simulink model "consigna_5_2"  (R2024b)
settings: Solver=ode45  StartTime=0.0  StopTime=600  FixedStep=1/39789  MaxStep=1e-1  RelTol=1e-5
InitFcn:
  | parametros
values from neighbouring files (symbols this model uses):
  A_corrientes = [0 1; -omega_n_corrientes^2 -2*omega_n_corrientes]    [parametros.m]
  A_inversor = [0 1; -omega_n_inversor^2 -2*omega_n_inversor]    [parametros.m]
  A_posicion = [0 1; -omega_n_posicion^2 -2*omega_n_posicion]    [parametros.m]
  A_temp = -1/20    (= -0.05)    [parametros.m]
  alpha_cu = 3.9 *10^-3    (= 0.0039)    [parametros.m]
  B_corrientes = [0; omega_n_corrientes^2]    [parametros.m]
  B_inversor = [0; omega_n_inversor^2]    [parametros.m]
  b_l = 0.1    [parametros.m]
  b_m = 1.5 * 10^-5    (= 1.5e-05)    [parametros.m]
  B_posicion = [0; omega_n_posicion^2]    [parametros.m]
  B_temp = 1/20    (= 0.05)    [parametros.m]
  ba = J_eq*n*omega_pos    (= 0.0395694444444)    [parametros.m]
  C_corrientes = [1 0]    [parametros.m]
  C_inversor = [1 0]    [parametros.m]
  C_posicion = [1 0]    [parametros.m]
  C_temp = 1    [parametros.m]
  C_ts = 0.818    [parametros.m]
  J_l = (m*l_cm^2 + J_cm) + (m_l * l_l^2)    (= 0.0833)    [parametros.m]
  J_m = 1.4 * 10^-5    (= 1.4e-05)    [parametros.m]
  K_e_int = 3200 ^3    (= 32768000000)    [parametros.m]
  K_e_omega = 3*3200^2    (= 30720000)    [parametros.m]
  K_e_theta = 9600    [parametros.m]
  k_l = m * g * l_cm + m_l * g * l_l    (= 2.4516625)    [parametros.m]
  Ksa = J_eq*n*(omega_pos^2)    (= 31.6555555556)    [parametros.m]
  Ksia = J_eq*(omega_pos^3)    (= 10129.7777778)    [parametros.m]
  L_d = 6.6 * 10^-3    (= 0.0066)    [parametros.m]
  L_ls = 0.8 * 10^-3    (= 0.0008)    [parametros.m]
  L_q = 5.8 * 10^-3    (= 0.0058)    [parametros.m]
  lambda_m = 0.016    [parametros.m]
  P_p = 3    [parametros.m]
  r = 120    [parametros.m]
  R_s_40 = 1.02    [parametros.m]
  R_ts_amb = 146.7    [parametros.m]
  T_sample = 1/f_sample    (= 4.53514739229e-05)    [parametros.m]
  Temp_s_ref = 20    [parametros.m]
  tm = X(1)    [parametros.m]
  tr = X(2)    [parametros.m]
  w1 = 2*pi*r/5    (= 150.796447372)    [parametros.m]
  x0_corrientes = [0;0]    [parametros.m]
  x0_inversor = [0;0]    [parametros.m]
  x0_posicion = [0; 0]    [parametros.m]
  x0_temp = 25    [parametros.m]
libraries: simulink x23, dspsigops x6
(part 5 of 5)

== system consigna_5_2/Subsystem/5.2.6/Subsistema físico no lineal ==
  note: Retroalimentación natural del torque gravitacional
  T_per : Inport
  v_as : Inport  Port=2
  v_bs : Inport  Port=3
  v_cs : Inport  Port=4
  Tº_amb : Inport  Port=5
  Gain : Gain  Gain=P_p
  Gain1 : Gain  Gain=1/r
  Gain2 : Gain  Gain=k_l
  Mux : Mux  Inputs=3
  Scope : Scope
  Sin : Trigonometry
  Subsistema electromagnético : Subsystem
      settings: PortSchema="{\"entries\":[{\"content\":{\"sides\":[{\"content\":{\"connectorIds\":[\"In1\",\"In2\",\"In3\",\"In4\"]},\"type\":\"ConnectorPlacement.EquallySpacedRectSide\",\"uuid\":\"c9fae60f-a644-4c7d-9a50-e330e891aba8\"},{\"content\":{\"connectorIds\":[\"Out1\",\"Out2\",\"Out3\",\"Out4\"],\"side\":\"RIGHT\"},\"type\":\"ConnectorPlacement.EquallySpacedRectSide\",\"uuid\":\"1bd25713-f5e9-4106-83eb-fb9f8a30d88e\"},{\"content\":{\"connectorIds\":[\"In5\"],\"side\":\"TOP\"},\"type\":\"ConnectorPlacement.EquallySpacedRectSide\",\"uuid\":\"c2f005dd-e04f-426d-b804-ce475aa5422d\"}]},\"type\":\"ConnectorPlacement.EquallySpacedConnector\",\"uuid\":\"9bdc4406-fcef-47cb-a5c0-d4f33f547a91\"}],\"packageUris\":[\"http://schema.mathworks.com/mf0/Connector/R2020b\"],\"version\":\"1.0\"}"
  Subsistema mecánico completo : Subsystem
  Subsistema térmico : Subsystem
  Sum : Sum  Inputs=++|
  TD_PARK : MATLAB Function  TreatAsAtomicUnit=on
  TI_PARK : MATLAB Function  TreatAsAtomicUnit=on
  theta_m : Outport
  T_s : Outport  Port=2
  i_abcs : Outport  Port=3
  omega_m : Outport  Port=4
  T_m : Outport  Port=5
  T_l : Outport  Port=6
  wires:
  Subsistema electromagnético/4(T_m) -> T_m/1, Subsistema mecánico completo/1(T_m)
  Subsistema electromagnético/3(i_0s) -> Subsistema térmico/3(i_0s^r), TI_PARK/3(f0s)
  Subsistema mecánico completo/2(omega_m(t)) -> Subsistema electromagnético/5(omega_m), Scope/1, omega_m/1
  Subsistema electromagnético/1(i_qs^r) -> Subsistema térmico/1(i_qs^r), TI_PARK/1(fqs)
  Subsistema electromagnético/2(i_ds^r) -> Subsistema térmico/2(i_ds^r), TI_PARK/2(fds)
  Sum/1 -> T_l/1, Subsistema mecánico completo/2(T_l)  "T_l"
  TD_PARK/1(fqs) -> Subsistema electromagnético/1(v_qs^r)
  Tº_amb/1 -> Subsistema térmico/4(Tº_amb)
  Mux/1 -> i_abcs/1
  TI_PARK/1(fas) -> Mux/1
  TI_PARK/2(fbs) -> Mux/2
  TI_PARK/3(fcs) -> Mux/3
  v_as/1 -> TD_PARK/1(fas)
  v_cs/1 -> TD_PARK/3(fcs)
  Gain/1 -> TI_PARK/4(theta_r), TD_PARK/4(theta_r)
  v_bs/1 -> TD_PARK/2(fbs)
  Gain1/1 -> Sin/1
  Sin/1 -> Gain2/1
  Gain2/1 -> Sum/1
  T_per/1 -> Sum/2
  TD_PARK/2(fds) -> Subsistema electromagnético/2(v_ds^r)
  TD_PARK/3(f0s) -> Subsistema electromagnético/3(v_0s)
  Subsistema térmico/1(r_s) -> Subsistema electromagnético/4(r_s)
  Subsistema térmico/2(T_s) -> T_s/1
  Subsistema mecánico completo/1(theta_m(t)) -> theta_m/1, Gain1/1, Gain/1

== system consigna_5_2/Subsystem/5.2.6/Controlador PID/Integrador Discreto por Trapecios1 ==
  y : Inport
  Delay : Delay  DelayLength=1
  Delay One Step : Delay  DelayLength=1
  Gain : Gain  Gain=T_sample/2
  Sum : Sum  Inputs=++|
  Sum1 : Sum  Inputs=++|
  I : Outport
  wires:
  Gain/1 -> Sum1/2  "b"
  Sum/1 -> Gain/1  "c"
  Sum1/1 -> Delay/1, I/1  "a"
  y/1 -> Sum/2, Delay One Step/1
  Delay/1 -> Sum1/1
  Delay One Step/1 -> Sum/1

== system consigna_5_2/Subsystem/5.2.6/Controlador PID/Integrador Discreto por Trapecios2 ==
  y : Inport
  Delay : Delay  DelayLength=1
  Delay One Step : Delay  DelayLength=1
  Gain : Gain  Gain=T_sample/2
  Sum : Sum  Inputs=++|
  Sum1 : Sum  Inputs=++|
  I : Outport
  wires:
  Gain/1 -> Sum1/2  "b"
  Sum/1 -> Gain/1  "c"
  Sum1/1 -> Delay/1, I/1  "a"
  y/1 -> Sum/2, Delay One Step/1
  Delay/1 -> Sum1/1
  Delay One Step/1 -> Sum/1

== system consigna_5_2/Subsystem/5.2.6/Observador de estado reducido/Integrador Discreto por Trapecios1 ==
  y : Inport
  Delay : Delay  DelayLength=1
  Delay One Step : Delay  DelayLength=1
  Gain : Gain  Gain=T_sample/2
  Sum : Sum  Inputs=++|
  Sum1 : Sum  Inputs=++|
  I : Outport
  wires:
  Delay One Step/1 -> Sum/1
  Sum/1 -> Gain/1  "c"
  Gain/1 -> Sum1/2  "b"
  y/1 -> Sum/2, Delay One Step/1
  Sum1/1 -> Delay/1, I/1  "a"
  Delay/1 -> Sum1/1

== system consigna_5_2/Subsystem/5.2.6/Observador de estado reducido/Integrador Discreto por Trapecios2 ==
  y : Inport
  Delay : Delay  DelayLength=1
  Delay One Step : Delay  DelayLength=1
  Gain : Gain  Gain=T_sample/2
  Sum : Sum  Inputs=++|
  Sum1 : Sum  Inputs=++|
  I : Outport
  wires:
  Gain/1 -> Sum1/2  "b"
  Sum/1 -> Gain/1  "c"
  Sum1/1 -> Delay/1, I/1  "a"
  y/1 -> Sum/2, Delay One Step/1
  Delay/1 -> Sum1/1
  Delay One Step/1 -> Sum/1

== system consigna_5_2/Subsystem/5.2.6/Observador de estado reducido/Integrador Discreto por Trapecios3 ==
  u : Inport
  Delay : Delay  DelayLength=1
  Delay One Step : Delay  DelayLength=1
  Gain : Gain  Gain=T_sample/2
  Sum : Sum  Inputs=++|
  Sum1 : Sum  Inputs=++|
  I : Outport
  wires:
  Gain/1 -> Sum1/2  "b"
  Sum/1 -> Gain/1  "c"
  Sum1/1 -> Delay/1, I/1  "a"
  u/1 -> Sum/2, Delay One Step/1
  Delay/1 -> Sum1/1
  Delay One Step/1 -> Sum/1

== system consigna_5_2/Subsystem/5.2.6/Subsistema físico no lineal/Subsistema electromagnético ==
  v_qs^r : Inport
  v_ds^r : Inport  Port=2
  v_0s : Inport  Port=3
  r_s : Inport  Port=4
  omega_m : Inport  Port=5
  Gain : Gain  Gain=P_p
  Gain1 : Gain  Gain=L_d
  Gain2 : Gain  Gain=lambda_m
  Gain3 : Gain  Gain=1/L_q
  Gain4 : Gain  Gain=L_q
  Gain5 : Gain  Gain=1/L_d
  Gain6 : Gain  Gain=1/L_ls
  Gain7 : Gain  Gain=L_d-L_q
  Gain8 : Gain  Gain=lambda_m
  Gain9 : Gain  Gain=(3/2)*P_p
  Integrator : Integrator
  Integrator1 : Integrator
  Integrator2 : Integrator
  Product{,1..5} (6 alike) : Product
  Sum{,1..3,5} (5 alike) : Sum  Inputs=-+|
  Sum4 : Sum  Inputs=++|
  Sum6 : Sum  Inputs=++|
  i_qs^r : Outport
  i_ds^r : Outport  Port=2
  i_0s : Outport  Port=3
  T_m : Outport  Port=4
  wires:
  v_qs^r/1 -> Sum/2
  Product/1 -> Sum/1
  Sum/1 -> Sum1/2
  Integrator/1 -> Gain8/1, Product5/1, i_qs^r/1, Product/2, Gain4/1  "i_qs^r"
  omega_m/1 -> Gain/1
  Gain/1 -> Gain2/1, Product1/1, Product3/1
  Integrator1/1 -> Product2/2, Product5/2, i_ds^r/1, Gain1/1  "i_ds^r"
  Gain1/1 -> Product1/2
  Sum1/1 -> Sum2/2
  Sum2/1 -> Gain3/1
  Gain2/1 -> Sum2/1
  Product1/1 -> Sum1/1
  Gain3/1 -> Integrator/1
  Product2/1 -> Sum3/1
  v_ds^r/1 -> Sum3/2
  Sum3/1 -> Sum4/2
  Product3/1 -> Sum4/1
  Gain4/1 -> Product3/2
  Gain5/1 -> Integrator1/1
  Sum4/1 -> Gain5/1
  Integrator2/1 -> Product4/2, i_0s/1  "i_0s"
  r_s/1 -> Product4/1, Product/1, Product2/1
  Product4/1 -> Sum5/1
  v_0s/1 -> Sum5/2
  Sum5/1 -> Gain6/1
  Gain6/1 -> Integrator2/1
  Product5/1 -> Gain7/1
  Gain7/1 -> Sum6/2
  Gain8/1 -> Sum6/1
  Sum6/1 -> Gain9/1
  Gain9/1 -> T_m/1

== system consigna_5_2/Subsystem/5.2.6/Subsistema físico no lineal/Subsistema mecánico completo ==
  T_m : Inport
  T_l : Inport  Port=2
  Gain : Gain  Gain=b_m + b_l / (r^2)
  Gain1 : Gain  Gain=1/r
  Gain2 : Gain  Gain=1/(J_m + J_l / r^2)
  Sum : Sum  Inputs=-+-
  omega_m(0) = 0 : Integrator
  theta_m(0) = 0 : Integrator
  theta_m(t) : Outport
  omega_m(t) : Outport  Port=2
  wires:
  Gain2/1 -> omega_m(0) = 0/1  "domega_m(t)/dt"
  Gain1/1 -> Sum/1
  theta_m(0) = 0/1 -> theta_m(t)/1  "theta_m(t)"
  omega_m(0) = 0/1 -> omega_m(t)/1, Gain/1, theta_m(0) = 0/1  "omega_m(t)"
  Sum/1 -> Gain2/1
  Gain/1 -> Sum/3
  T_l/1 -> Gain1/1
  T_m/1 -> Sum/2

== system consigna_5_2/Subsystem/5.2.6/Subsistema físico no lineal/Subsistema térmico ==
  i_qs^r : Inport
  i_ds^r : Inport  Port=2
  i_0s^r : Inport  Port=3
  Tº_amb : Inport  Port=4
  Constant : Constant  Value=Temp_s_ref
  Constant1 : Constant
  Gain : Gain  Gain=1/C_ts
  Gain1 : Gain  Gain=3/2
  Gain2 : Gain  Gain=1/R_ts_amb
  Gain3 : Gain  Gain=alpha_cu
  Gain4 : Gain  Gain=R_s_40
  Gain5 : Gain  Gain=2
  Integrator : Integrator  InitialCondition=40
  Product : Product
  Square : Math  Operator=square
  Square1 : Math  Operator=square
  Square2 : Math  Operator=square
  Sum : Sum  Inputs=+++
  Sum1 : Sum  Inputs=-|+
  Sum2 : Sum  Inputs=|+-
  Sum3 : Sum  Inputs=|+-
  Sum4 : Sum  Inputs=|++
  r_s : Outport
  T_s : Outport  Port=2
  wires:
  i_qs^r/1 -> Square/1
  i_ds^r/1 -> Square1/1
  i_0s^r/1 -> Square2/1
  Gain/1 -> Integrator/1
  Square/1 -> Sum/1
  Square1/1 -> Sum/2
  Sum/1 -> Product/1
  Product/1 -> Gain1/1
  Tº_amb/1 -> Sum1/1
  Integrator/1 -> T_s/1, Sum3/1, Sum1/2
  Sum1/1 -> Gain2/1
  Gain1/1 -> Sum2/1
  Gain2/1 -> Sum2/2
  Sum2/1 -> Gain/1
  Constant/1 -> Sum3/2
  Sum3/1 -> Gain3/1
  Gain3/1 -> Sum4/1
  Constant1/1 -> Sum4/2
  Sum4/1 -> Gain4/1
  Gain4/1 -> Product/2, r_s/1
  Square2/1 -> Gain5/1
  Gain5/1 -> Sum/3

== matlab function consigna_5_2/5.2.4.b/TD_PARK ==
  data: fas input; fqs output; fbs input; fcs input; theta_r input; fds output; f0s output
function [fqs, fds, f0s] = TD_PARK(fas, fbs, fcs, theta_r)

    fabcs = [fas; fbs; fcs];

    Ks = 2/3*[cos(theta_r) cos(theta_r - 2*pi/3) cos(theta_r + 2*pi/3)
          sin(theta_r) sin(theta_r - 2*pi/3) sin(theta_r + 2*pi/3) 
          1/2          1/2                   1/2];

    fqd0s = Ks * fabcs;

    fqs = fqd0s(1);
    fds = fqd0s(2);
    f0s = fqd0s(3);

end

== matlab function consigna_5_2/5.2.4.b/TI_PARK1 ==
  data: fqs input; fas output; fds input; f0s input; theta_r input; fbs output; fcs output
function [fas, fbs, fcs] = TI_PARK(fqs, fds, f0s , theta_r)

    fqd0s = [fqs; fds; f0s];

    Ks = [cos(theta_r)         sin(theta_r)             1
          cos(theta_r - 2*pi/3) sin(theta_r - 2*pi/3)    1
          cos(theta_r + 2*pi/3) sin(theta_r + 2*pi/3)    1];

    fabcs = Ks * fqd0s;

    fas = fabcs(1);
    fbs = fabcs(2);
    fcs = fabcs(3);

end

== matlab function consigna_5_2/5.2.1 /Subsistema físico no lineal/TD_PARK ==
  data: fas input; fqs output; fbs input; fcs input; theta_r input; fds output; f0s output
function [fqs, fds, f0s] = TD_PARK(fas, fbs, fcs, theta_r)

    fabcs = [fas; fbs; fcs];

    Ks = 2/3*[cos(theta_r) cos(theta_r - 2*pi/3) cos(theta_r + 2*pi/3)
          sin(theta_r) sin(theta_r - 2*pi/3) sin(theta_r + 2*pi/3) 
          1/2          1/2                   1/2];

    fqd0s = Ks * fabcs;

    fqs = fqd0s(1);
    fds = fqd0s(2);
    f0s = fqd0s(3);

end

== matlab function consigna_5_2/5.2.3/Subsistema físico no lineal/TD_PARK ==
  data: fas input; fqs output; fbs input; fcs input; theta_r input; fds output; f0s output
function [fqs, fds, f0s] = TD_PARK(fas, fbs, fcs, theta_r)

    fabcs = [fas; fbs; fcs];

    Ks = 2/3*[cos(theta_r) cos(theta_r - 2*pi/3) cos(theta_r + 2*pi/3)
          sin(theta_r) sin(theta_r - 2*pi/3) sin(theta_r + 2*pi/3) 
          1/2          1/2                   1/2];

    fqd0s = Ks * fabcs;

    fqs = fqd0s(1);
    fds = fqd0s(2);
    f0s = fqd0s(3);

end

== matlab function consigna_5_2/5.2.3/Subsistema físico no lineal/TI_PARK ==
  data: fqs input; fas output; fds input; f0s input; theta_r input; fbs output; fcs output
function [fas, fbs, fcs] = TI_PARK(fqs, fds, f0s , theta_r)

    fqd0s = [fqs; fds; f0s];

    Ks = [cos(theta_r)         sin(theta_r)             1
          cos(theta_r - 2*pi/3) sin(theta_r - 2*pi/3)    1
          cos(theta_r + 2*pi/3) sin(theta_r + 2*pi/3)    1];

    fabcs = Ks * fqd0s;

    fas = fabcs(1);
    fbs = fabcs(2);
    fcs = fabcs(3);

end

== matlab function consigna_5_2/5.2.5/Subsistema físico no lineal/TD_PARK ==
  data: fas input; fqs output; fbs input; fcs input; theta_r input; fds output; f0s output
function [fqs, fds, f0s] = TD_PARK(fas, fbs, fcs, theta_r)

    fabcs = [fas; fbs; fcs];

    Ks = 2/3*[cos(theta_r) cos(theta_r - 2*pi/3) cos(theta_r + 2*pi/3)
          sin(theta_r) sin(theta_r - 2*pi/3) sin(theta_r + 2*pi/3) 
          1/2          1/2                   1/2];

    fqd0s = Ks * fabcs;

    fqs = fqd0s(1);
    fds = fqd0s(2);
    f0s = fqd0s(3);

end

== matlab function consigna_5_2/5.2.5/Subsistema físico no lineal/TI_PARK ==
  data: fqs input; fas output; fds input; f0s input; theta_r input; fbs output; fcs output
function [fas, fbs, fcs] = TI_PARK(fqs, fds, f0s , theta_r)

    fqd0s = [fqs; fds; f0s];

    Ks = [cos(theta_r)         sin(theta_r)             1
          cos(theta_r - 2*pi/3) sin(theta_r - 2*pi/3)    1
          cos(theta_r + 2*pi/3) sin(theta_r + 2*pi/3)    1];

    fabcs = Ks * fqd0s;

    fas = fabcs(1);
    fbs = fabcs(2);
    fcs = fabcs(3);

end

== matlab function consigna_5_2/5.2.5/TD_PARK ==
  data: fas input; fqs output; fbs input; fcs input; theta_r input; fds output; f0s output
function [fqs, fds, f0s] = TD_PARK(fas, fbs, fcs, theta_r)

    fabcs = [fas; fbs; fcs];

    Ks = 2/3*[cos(theta_r) cos(theta_r - 2*pi/3) cos(theta_r + 2*pi/3)
          sin(theta_r) sin(theta_r - 2*pi/3) sin(theta_r + 2*pi/3) 
          1/2          1/2                   1/2];

    fqd0s = Ks * fabcs;

    fqs = fqd0s(1);
    fds = fqd0s(2);
    f0s = fqd0s(3);

end

== matlab function consigna_5_2/5.2.5/TI_PARK1 ==
  data: fqs input; fas output; fds input; f0s input; theta_r input; fbs output; fcs output
function [fas, fbs, fcs] = TI_PARK(fqs, fds, f0s , theta_r)

    fqd0s = [fqs; fds; f0s];

    Ks = [cos(theta_r)         sin(theta_r)             1
          cos(theta_r - 2*pi/3) sin(theta_r - 2*pi/3)    1
          cos(theta_r + 2*pi/3) sin(theta_r + 2*pi/3)    1];

    fabcs = Ks * fqd0s;

    fas = fabcs(1);
    fbs = fabcs(2);
    fcs = fabcs(3);

end

== matlab function consigna_5_2/5.2.5'/Subsistema físico no lineal/TD_PARK ==
  data: fas input; fqs output; fbs input; fcs input; theta_r input; fds output; f0s output
function [fqs, fds, f0s] = TD_PARK(fas, fbs, fcs, theta_r)

    fabcs = [fas; fbs; fcs];

    Ks = 2/3*[cos(theta_r) cos(theta_r - 2*pi/3) cos(theta_r + 2*pi/3)
          sin(theta_r) sin(theta_r - 2*pi/3) sin(theta_r + 2*pi/3) 
          1/2          1/2                   1/2];

    fqd0s = Ks * fabcs;

    fqs = fqd0s(1);
    fds = fqd0s(2);
    f0s = fqd0s(3);

end

== matlab function consigna_5_2/5.2.5'/Subsistema físico no lineal/TI_PARK ==
  data: fqs input; fas output; fds input; f0s input; theta_r input; fbs output; fcs output
function [fas, fbs, fcs] = TI_PARK(fqs, fds, f0s , theta_r)

    fqd0s = [fqs; fds; f0s];

    Ks = [cos(theta_r)         sin(theta_r)             1
          cos(theta_r - 2*pi/3) sin(theta_r - 2*pi/3)    1
          cos(theta_r + 2*pi/3) sin(theta_r + 2*pi/3)    1];

    fabcs = Ks * fqd0s;

    fas = fabcs(1);
    fbs = fabcs(2);
    fcs = fabcs(3);

end

== matlab function consigna_5_2/5.2.5'/TD_PARK ==
  data: fas input; fqs output; fbs input; fcs input; theta_r input; fds output; f0s output
function [fqs, fds, f0s] = TD_PARK(fas, fbs, fcs, theta_r)

    fabcs = [fas; fbs; fcs];

    Ks = 2/3*[cos(theta_r) cos(theta_r - 2*pi/3) cos(theta_r + 2*pi/3)
          sin(theta_r) sin(theta_r - 2*pi/3) sin(theta_r + 2*pi/3) 
          1/2          1/2                   1/2];

    fqd0s = Ks * fabcs;

    fqs = fqd0s(1);
    fds = fqd0s(2);
    f0s = fqd0s(3);

end

== matlab function consigna_5_2/5.2.5'/TI_PARK1 ==
  data: fqs input; fas output; fds input; f0s input; theta_r input; fbs output; fcs output
function [fas, fbs, fcs] = TI_PARK(fqs, fds, f0s , theta_r)

    fqd0s = [fqs; fds; f0s];

    Ks = [cos(theta_r)         sin(theta_r)             1
          cos(theta_r - 2*pi/3) sin(theta_r - 2*pi/3)    1
          cos(theta_r + 2*pi/3) sin(theta_r + 2*pi/3)    1];

    fabcs = Ks * fqd0s;

    fas = fabcs(1);
    fbs = fabcs(2);
    fcs = fabcs(3);

end

== matlab function consigna_5_2/5.2.1 /Subsistema físico no lineal/TI_PARK ==
  data: fqs input; fas output; fds input; f0s input; theta_r input; fbs output; fcs output
function [fas, fbs, fcs] = TI_PARK(fqs, fds, f0s , theta_r)

    fqd0s = [fqs; fds; f0s];

    Ks = [cos(theta_r)         sin(theta_r)             1
          cos(theta_r - 2*pi/3) sin(theta_r - 2*pi/3)    1
          cos(theta_r + 2*pi/3) sin(theta_r + 2*pi/3)    1];

    fabcs = Ks * fqd0s;

    fas = fabcs(1);
    fbs = fabcs(2);
    fcs = fabcs(3);

end

== matlab function consigna_5_2/5.2.5.c/Subsistema físico no lineal/TD_PARK ==
  data: fas input; fqs output; fbs input; fcs input; theta_r input; fds output; f0s output
function [fqs, fds, f0s] = TD_PARK(fas, fbs, fcs, theta_r)

    fabcs = [fas; fbs; fcs];

    Ks = 2/3*[cos(theta_r) cos(theta_r - 2*pi/3) cos(theta_r + 2*pi/3)
          sin(theta_r) sin(theta_r - 2*pi/3) sin(theta_r + 2*pi/3) 
          1/2          1/2                   1/2];

    fqd0s = Ks * fabcs;

    fqs = fqd0s(1);
    fds = fqd0s(2);
    f0s = fqd0s(3);

end

== matlab function consigna_5_2/5.2.5.c/Subsistema físico no lineal/TI_PARK ==
  data: fqs input; fas output; fds input; f0s input; theta_r input; fbs output; fcs output
function [fas, fbs, fcs] = TI_PARK(fqs, fds, f0s , theta_r)

    fqd0s = [fqs; fds; f0s];

    Ks = [cos(theta_r)         sin(theta_r)             1
          cos(theta_r - 2*pi/3) sin(theta_r - 2*pi/3)    1
          cos(theta_r + 2*pi/3) sin(theta_r + 2*pi/3)    1];

    fabcs = Ks * fqd0s;

    fas = fabcs(1);
    fbs = fabcs(2);
    fcs = fabcs(3);

end

== matlab function consigna_5_2/5.2.5.c/TD_PARK ==
  data: fas input; fqs output; fbs input; fcs input; theta_r input; fds output; f0s output
function [fqs, fds, f0s] = TD_PARK(fas, fbs, fcs, theta_r)

    fabcs = [fas; fbs; fcs];

    Ks = 2/3*[cos(theta_r) cos(theta_r - 2*pi/3) cos(theta_r + 2*pi/3)
          sin(theta_r) sin(theta_r - 2*pi/3) sin(theta_r + 2*pi/3) 
          1/2          1/2                   1/2];

    fqd0s = Ks * fabcs;

    fqs = fqd0s(1);
    fds = fqd0s(2);
    f0s = fqd0s(3);

end

== matlab function consigna_5_2/5.2.5.c/TI_PARK1 ==
  data: fqs input; fas output; fds input; f0s input; theta_r input; fbs output; fcs output
function [fas, fbs, fcs] = TI_PARK(fqs, fds, f0s , theta_r)

    fqd0s = [fqs; fds; f0s];

    Ks = [cos(theta_r)         sin(theta_r)             1
          cos(theta_r - 2*pi/3) sin(theta_r - 2*pi/3)    1
          cos(theta_r + 2*pi/3) sin(theta_r + 2*pi/3)    1];

    fabcs = Ks * fqd0s;

    fas = fabcs(1);
    fbs = fabcs(2);
    fcs = fabcs(3);

end

== matlab function consigna_5_2/5.2.5.d/Subsistema físico no lineal/TD_PARK ==
  data: fas input; fqs output; fbs input; fcs input; theta_r input; fds output; f0s output
function [fqs, fds, f0s] = TD_PARK(fas, fbs, fcs, theta_r)

    fabcs = [fas; fbs; fcs];

    Ks = 2/3*[cos(theta_r) cos(theta_r - 2*pi/3) cos(theta_r + 2*pi/3)
          sin(theta_r) sin(theta_r - 2*pi/3) sin(theta_r + 2*pi/3) 
          1/2          1/2                   1/2];

    fqd0s = Ks * fabcs;

    fqs = fqd0s(1);
    fds = fqd0s(2);
    f0s = fqd0s(3);

end

== matlab function consigna_5_2/5.2.5.d/Subsistema físico no lineal/TI_PARK ==
  data: fqs input; fas output; fds input; f0s input; theta_r input; fbs output; fcs output
function [fas, fbs, fcs] = TI_PARK(fqs, fds, f0s , theta_r)

    fqd0s = [fqs; fds; f0s];

    Ks = [cos(theta_r)         sin(theta_r)             1
          cos(theta_r - 2*pi/3) sin(theta_r - 2*pi/3)    1
          cos(theta_r + 2*pi/3) sin(theta_r + 2*pi/3)    1];

    fabcs = Ks * fqd0s;

    fas = fabcs(1);
    fbs = fabcs(2);
    fcs = fabcs(3);

end

== matlab function consigna_5_2/5.2.5.d/TD_PARK ==
  data: fas input; fqs output; fbs input; fcs input; theta_r input; fds output; f0s output
function [fqs, fds, f0s] = TD_PARK(fas, fbs, fcs, theta_r)

    fabcs = [fas; fbs; fcs];

    Ks = 2/3*[cos(theta_r) cos(theta_r - 2*pi/3) cos(theta_r + 2*pi/3)
          sin(theta_r) sin(theta_r - 2*pi/3) sin(theta_r + 2*pi/3) 
          1/2          1/2                   1/2];

    fqd0s = Ks * fabcs;

    fqs = fqd0s(1);
    fds = fqd0s(2);
    f0s = fqd0s(3);

end

== matlab function consigna_5_2/5.2.5.d/TI_PARK1 ==
  data: fqs input; fas output; fds input; f0s input; theta_r input; fbs output; fcs output
function [fas, fbs, fcs] = TI_PARK(fqs, fds, f0s , theta_r)

    fqd0s = [fqs; fds; f0s];

    Ks = [cos(theta_r)         sin(theta_r)             1
          cos(theta_r - 2*pi/3) sin(theta_r - 2*pi/3)    1
          cos(theta_r + 2*pi/3) sin(theta_r + 2*pi/3)    1];

    fabcs = Ks * fqd0s;

    fas = fabcs(1);
    fbs = fabcs(2);
    fcs = fabcs(3);

end

== matlab function consigna_5_2/5.2.5.e/Subsistema físico no lineal/TD_PARK ==
  data: fas input; fqs output; fbs input; fcs input; theta_r input; fds output; f0s output
function [fqs, fds, f0s] = TD_PARK(fas, fbs, fcs, theta_r)

    fabcs = [fas; fbs; fcs];

    Ks = 2/3*[cos(theta_r) cos(theta_r - 2*pi/3) cos(theta_r + 2*pi/3)
          sin(theta_r) sin(theta_r - 2*pi/3) sin(theta_r + 2*pi/3) 
          1/2          1/2                   1/2];

    fqd0s = Ks * fabcs;

    fqs = fqd0s(1);
    fds = fqd0s(2);
    f0s = fqd0s(3);

end

== matlab function consigna_5_2/5.2.5.e/Subsistema físico no lineal/TI_PARK ==
  data: fqs input; fas output; fds input; f0s input; theta_r input; fbs output; fcs output
function [fas, fbs, fcs] = TI_PARK(fqs, fds, f0s , theta_r)

    fqd0s = [fqs; fds; f0s];

    Ks = [cos(theta_r)         sin(theta_r)             1
          cos(theta_r - 2*pi/3) sin(theta_r - 2*pi/3)    1
          cos(theta_r + 2*pi/3) sin(theta_r + 2*pi/3)    1];

    fabcs = Ks * fqd0s;

    fas = fabcs(1);
    fbs = fabcs(2);
    fcs = fabcs(3);

end

== matlab function consigna_5_2/5.2.4/Subsistema físico no lineal/TD_PARK ==
  data: fas input; fqs output; fbs input; fcs input; theta_r input; fds output; f0s output
function [fqs, fds, f0s] = TD_PARK(fas, fbs, fcs, theta_r)

    fabcs = [fas; fbs; fcs];

    Ks = 2/3*[cos(theta_r) cos(theta_r - 2*pi/3) cos(theta_r + 2*pi/3)
          sin(theta_r) sin(theta_r - 2*pi/3) sin(theta_r + 2*pi/3) 
          1/2          1/2                   1/2];

    fqd0s = Ks * fabcs;

    fqs = fqd0s(1);
    fds = fqd0s(2);
    f0s = fqd0s(3);

end

== matlab function consigna_5_2/5.2.5.e/TD_PARK ==
  data: fas input; fqs output; fbs input; fcs input; theta_r input; fds output; f0s output
function [fqs, fds, f0s] = TD_PARK(fas, fbs, fcs, theta_r)

    fabcs = [fas; fbs; fcs];

    Ks = 2/3*[cos(theta_r) cos(theta_r - 2*pi/3) cos(theta_r + 2*pi/3)
          sin(theta_r) sin(theta_r - 2*pi/3) sin(theta_r + 2*pi/3) 
          1/2          1/2                   1/2];

    fqd0s = Ks * fabcs;

    fqs = fqd0s(1);
    fds = fqd0s(2);
    f0s = fqd0s(3);

end

== matlab function consigna_5_2/5.2.5.e/TI_PARK1 ==
  data: fqs input; fas output; fds input; f0s input; theta_r input; fbs output; fcs output
function [fas, fbs, fcs] = TI_PARK(fqs, fds, f0s , theta_r)

    fqd0s = [fqs; fds; f0s];

    Ks = [cos(theta_r)         sin(theta_r)             1
          cos(theta_r - 2*pi/3) sin(theta_r - 2*pi/3)    1
          cos(theta_r + 2*pi/3) sin(theta_r + 2*pi/3)    1];

    fabcs = Ks * fqd0s;

    fas = fabcs(1);
    fbs = fabcs(2);
    fcs = fabcs(3);

end

== matlab function consigna_5_2/5.2.1 /TI_PARK1 ==
  data: fqs input; fas output; fds input; f0s input; theta_r input; fbs output; fcs output
function [fas, fbs, fcs] = TI_PARK(fqs, fds, f0s , theta_r)

    fqd0s = [fqs; fds; f0s];

    Ks = [cos(theta_r)         sin(theta_r)             1
          cos(theta_r - 2*pi/3) sin(theta_r - 2*pi/3)    1
          cos(theta_r + 2*pi/3) sin(theta_r + 2*pi/3)    1];

    fabcs = Ks * fqd0s;

    fas = fabcs(1);
    fbs = fabcs(2);
    fcs = fabcs(3);

end

== matlab function consigna_5_2/5.2.1 /TD_PARK ==
  data: fas input; fqs output; fbs input; fcs input; theta_r input; fds output; f0s output
function [fqs, fds, f0s] = TD_PARK(fas, fbs, fcs, theta_r)

    fabcs = [fas; fbs; fcs];

    Ks = 2/3*[cos(theta_r) cos(theta_r - 2*pi/3) cos(theta_r + 2*pi/3)
          sin(theta_r) sin(theta_r - 2*pi/3) sin(theta_r + 2*pi/3) 
          1/2          1/2                   1/2];

    fqd0s = Ks * fabcs;

    fqs = fqd0s(1);
    fds = fqd0s(2);
    f0s = fqd0s(3);

end

== matlab function consigna_5_2/MATLAB Function ==
  data: y output; t input
function y = fcn(t)

while t>20
    t = t - 20;
end

if t <= 5

    y = 2*pi*t/5;

elseif t <= 10

    y = 2*pi;

elseif t <= 15

    y = 2*pi-2*pi*(t-10)/5;

else 

    y = 0;

end

== matlab function consigna_5_2/Subsystem/5.2.6/Subsistema físico no lineal/TD_PARK ==
  data: fas input; fqs output; fbs input; fcs input; theta_r input; fds output; f0s output
function [fqs, fds, f0s] = TD_PARK(fas, fbs, fcs, theta_r)

    fabcs = [fas; fbs; fcs];

    Ks = 2/3*[cos(theta_r) cos(theta_r - 2*pi/3) cos(theta_r + 2*pi/3)
          sin(theta_r) sin(theta_r - 2*pi/3) sin(theta_r + 2*pi/3) 
          1/2          1/2                   1/2];

    fqd0s = Ks * fabcs;

    fqs = fqd0s(1);
    fds = fqd0s(2);
    f0s = fqd0s(3);

end

== matlab function consigna_5_2/5.2.3/TD_PARK ==
  data: fas input; fqs output; fbs input; fcs input; theta_r input; fds output; f0s output
function [fqs, fds, f0s] = TD_PARK(fas, fbs, fcs, theta_r)

    fabcs = [fas; fbs; fcs];

    Ks = 2/3*[cos(theta_r) cos(theta_r - 2*pi/3) cos(theta_r + 2*pi/3)
          sin(theta_r) sin(theta_r - 2*pi/3) sin(theta_r + 2*pi/3) 
          1/2          1/2                   1/2];

    fqd0s = Ks * fabcs;

    fqs = fqd0s(1);
    fds = fqd0s(2);
    f0s = fqd0s(3);

end

== matlab function consigna_5_2/5.2.3/TI_PARK1 ==
  data: fqs input; fas output; fds input; f0s input; theta_r input; fbs output; fcs output
function [fas, fbs, fcs] = TI_PARK(fqs, fds, f0s , theta_r)

    fqd0s = [fqs; fds; f0s];

    Ks = [cos(theta_r)         sin(theta_r)             1
          cos(theta_r - 2*pi/3) sin(theta_r - 2*pi/3)    1
          cos(theta_r + 2*pi/3) sin(theta_r + 2*pi/3)    1];

    fabcs = Ks * fqd0s;

    fas = fabcs(1);
    fbs = fabcs(2);
    fcs = fabcs(3);

end

== matlab function consigna_5_2/Subsystem/5.2.6/Subsistema físico no lineal/TI_PARK ==
  data: fqs input; fas output; fds input; f0s input; theta_r input; fbs output; fcs output
function [fas, fbs, fcs] = TI_PARK(fqs, fds, f0s , theta_r)

    fqd0s = [fqs; fds; f0s];

    Ks = [cos(theta_r)         sin(theta_r)             1
          cos(theta_r - 2*pi/3) sin(theta_r - 2*pi/3)    1
          cos(theta_r + 2*pi/3) sin(theta_r + 2*pi/3)    1];

    fabcs = Ks * fqd0s;

    fas = fabcs(1);
    fbs = fabcs(2);
    fcs = fabcs(3);

end

== matlab function consigna_5_2/Subsystem/5.2.6/TD_PARK ==
  data: fas input; fqs output; fbs input; fcs input; theta_r input; fds output; f0s output
function [fqs, fds, f0s] = TD_PARK(fas, fbs, fcs, theta_r)

    fabcs = [fas; fbs; fcs];

    Ks = 2/3*[cos(theta_r) cos(theta_r - 2*pi/3) cos(theta_r + 2*pi/3)
          sin(theta_r) sin(theta_r - 2*pi/3) sin(theta_r + 2*pi/3) 
          1/2          1/2                   1/2];

    fqd0s = Ks * fabcs;

    fqs = fqd0s(1);
    fds = fqd0s(2);
    f0s = fqd0s(3);

end

== matlab function consigna_5_2/Subsystem/5.2.6/TI_PARK1 ==
  data: fqs input; fas output; fds input; f0s input; theta_r input; fbs output; fcs output
function [fas, fbs, fcs] = TI_PARK(fqs, fds, f0s , theta_r)

    fqd0s = [fqs; fds; f0s];

    Ks = [cos(theta_r)         sin(theta_r)             1
          cos(theta_r - 2*pi/3) sin(theta_r - 2*pi/3)    1
          cos(theta_r + 2*pi/3) sin(theta_r + 2*pi/3)    1];

    fabcs = Ks * fqd0s;

    fas = fabcs(1);
    fbs = fabcs(2);
    fcs = fabcs(3);

end

== matlab function consigna_5_2/5.2.4/Subsistema físico no lineal/TI_PARK ==
  data: fqs input; fas output; fds input; f0s input; theta_r input; fbs output; fcs output
function [fas, fbs, fcs] = TI_PARK(fqs, fds, f0s , theta_r)

    fqd0s = [fqs; fds; f0s];

    Ks = [cos(theta_r)         sin(theta_r)             1
          cos(theta_r - 2*pi/3) sin(theta_r - 2*pi/3)    1
          cos(theta_r + 2*pi/3) sin(theta_r + 2*pi/3)    1];

    fabcs = Ks * fqd0s;

    fas = fabcs(1);
    fbs = fabcs(2);
    fcs = fabcs(3);

end

== matlab function consigna_5_2/5.2.4/TD_PARK ==
  data: fas input; fqs output; fbs input; fcs input; theta_r input; fds output; f0s output
function [fqs, fds, f0s] = TD_PARK(fas, fbs, fcs, theta_r)

    fabcs = [fas; fbs; fcs];

    Ks = 2/3*[cos(theta_r) cos(theta_r - 2*pi/3) cos(theta_r + 2*pi/3)
          sin(theta_r) sin(theta_r - 2*pi/3) sin(theta_r + 2*pi/3) 
          1/2          1/2                   1/2];

    fqd0s = Ks * fabcs;

    fqs = fqd0s(1);
    fds = fqd0s(2);
    f0s = fqd0s(3);

end

== matlab function consigna_5_2/5.2.4/TI_PARK1 ==
  data: fqs input; fas output; fds input; f0s input; theta_r input; fbs output; fcs output
function [fas, fbs, fcs] = TI_PARK(fqs, fds, f0s , theta_r)

    fqd0s = [fqs; fds; f0s];

    Ks = [cos(theta_r)         sin(theta_r)             1
          cos(theta_r - 2*pi/3) sin(theta_r - 2*pi/3)    1
          cos(theta_r + 2*pi/3) sin(theta_r + 2*pi/3)    1];

    fabcs = Ks * fqd0s;

    fas = fabcs(1);
    fbs = fabcs(2);
    fcs = fabcs(3);

end

== matlab function consigna_5_2/5.2.4.b/Subsistema físico no lineal/TD_PARK ==
  data: fas input; fqs output; fbs input; fcs input; theta_r input; fds output; f0s output
function [fqs, fds, f0s] = TD_PARK(fas, fbs, fcs, theta_r)

    fabcs = [fas; fbs; fcs];

    Ks = 2/3*[cos(theta_r) cos(theta_r - 2*pi/3) cos(theta_r + 2*pi/3)
          sin(theta_r) sin(theta_r - 2*pi/3) sin(theta_r + 2*pi/3) 
          1/2          1/2                   1/2];

    fqd0s = Ks * fabcs;

    fqs = fqd0s(1);
    fds = fqd0s(2);
    f0s = fqd0s(3);

end

== matlab function consigna_5_2/5.2.4.b/Subsistema físico no lineal/TI_PARK ==
  data: fqs input; fas output; fds input; f0s input; theta_r input; fbs output; fcs output
function [fas, fbs, fcs] = TI_PARK(fqs, fds, f0s , theta_r)

    fqd0s = [fqs; fds; f0s];

    Ks = [cos(theta_r)         sin(theta_r)             1
          cos(theta_r - 2*pi/3) sin(theta_r - 2*pi/3)    1
          cos(theta_r + 2*pi/3) sin(theta_r + 2*pi/3)    1];

    fabcs = Ks * fqd0s;

    fas = fabcs(1);
    fbs = fabcs(2);
    fcs = fabcs(3);

end
